simulink model "Cruise_control"  (R2018a)
settings: Solver=VariableStepAuto  StartTime=0.0  StopTime=10  MaxStep=0.01  RelTol=1e-4  EnableMultiTasking=on
values from neighbouring files (symbols this model uses):
  b_Ahead = 50    [ACC_DATA.m]    (also in CC_data.m)
  m_Ahead = 1000    [ACC_DATA.m]    (also in CC_data.m)
undefined symbols (not defined in the file or in its folder): b, m, sigbuilder_block
libraries: simulink x5
settings Model: Creator=Talha Rao  LastModifiedBy=Talha Rao
settings DataIOCC: LimitDataPoints=on  SaveOutput=off  SaveTime=off
settings OptimizationCC: ExpressionDepthLimit=2147483647  LifeSpan=1
settings DebuggingCC: UnderspecifiedInitializationDetection=Classic  MergeDetectMultiDrivingBlocksExec=none  FcnCallInpInsideContextMsg=warning  AllowSymbolicDim=off  StateNameClashWarn=warning  SFUnexpectedBacktrackingDiag=warning  SFNoUnconditionalDefaultTransitionDiag=warning  SFExecutionAtInitializationDiag=none
settings CodeAppCC: StateflowObjectComments=on
settings GRTTargetCC: TargetLangStandard=C89/C90 (ANSI)  GeneratePreprocessorConditionals=Disable all  CombineOutputUpdateFcns=off  GRTInterface=on

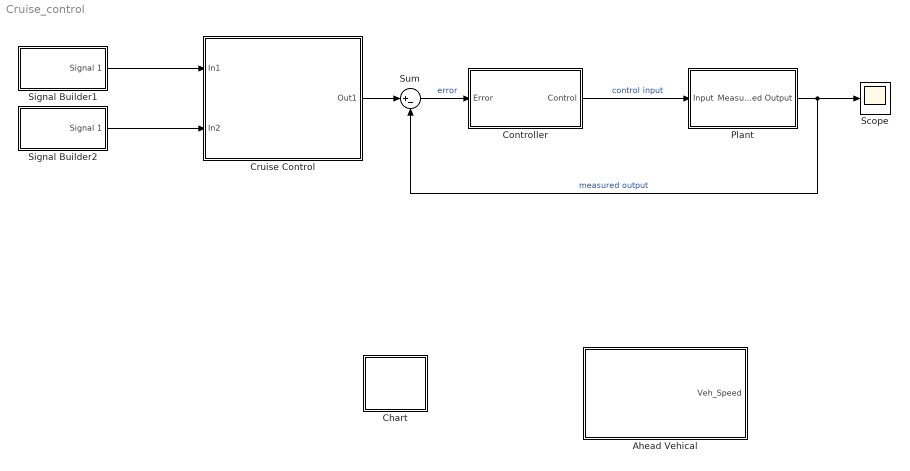
== system Cruise_control ==
  Ahead Vehical : Subsystem
      mask Display: image('C:\Users\Talha Rao\Pictures\index2 (2).jpg');
  Chart : Stateflow chart  TreatAsAtomicUnit=on
  Controller : Subsystem
  Cruise Control : Subsystem
  Plant : Subsystem
  Scope : Scope
  Signal Builder1 : Subsystem  Tag=STV Subsys  LoadFcn=sigbuilder_block('load');  StartFcn=sigbuilder_block('start');  StopFcn=sigbuilder_block('stop');  ClipboardFcn=sigbuilder_block('clipboard');  mask(Sigbuilder block){tuvar=[0:10]}
      mask help: Simulink:masks:SigbuilderBlock_MD
      mask init:
      | if ~strcmp(get_param(bdroot(gcbh),'SimulationStatus'),'stopped') tuvar = sigbuilder_block('maskInit'); end
      settings: CopyFcn=sigbuilder_block('copy');  DeleteFcn=sigbuilder_block('delete');  ModelCloseFcn=sigbuilder_block('modelClose');  PreSaveFcn=sigbuilder_block('preSave');  PauseFcn=sigbuilder_block('pause');  ContinueFcn=sigbuilder_block('continue');  NameChangeFcn=sigbuilder_block('namechange');  OpenFcn=sigbuilder_block('open',[437.6 199.2 550.4 400 ]);  CloseFcn=sigbuilder_block('close');
      mask Display: plot(0, 0, 100, 100,[2, 2, 32, 32, 2], [68, 8, 8, 68, 68],[32, 2], [38, 38], [32, 19, 2],[53, 60, 44], [32, 17, 17, 2],[16, 16, 31, 31]);txt = getActiveGroup(gcbh);text(2, 100, txt,'verticalAlignment', 'top');
  Signal Builder2 : Subsystem  Tag=STV Subsys  LoadFcn=sigbuilder_block('load');  StartFcn=sigbuilder_block('start');  StopFcn=sigbuilder_block('stop');  ClipboardFcn=sigbuilder_block('clipboard');  mask(Sigbuilder block){tuvar=[0:10]}
      mask help: Simulink:masks:SigbuilderBlock_MD
      mask init:
      | if ~strcmp(get_param(bdroot(gcbh),'SimulationStatus'),'stopped') tuvar = sigbuilder_block('maskInit'); end
      settings: CopyFcn=sigbuilder_block('copy');  DeleteFcn=sigbuilder_block('delete');  ModelCloseFcn=sigbuilder_block('modelClose');  PreSaveFcn=sigbuilder_block('preSave');  PauseFcn=sigbuilder_block('pause');  ContinueFcn=sigbuilder_block('continue');  NameChangeFcn=sigbuilder_block('namechange');  OpenFcn=sigbuilder_block('open',[437.6 199.2 550.4 400 ]);  CloseFcn=sigbuilder_block('close');
      mask Display: plot(0, 0, 100, 100,[2, 2, 32, 32, 2], [68, 8, 8, 68, 68],[32, 2], [38, 38], [32, 19, 2],[53, 60, 44], [32, 17, 17, 2],[16, 16, 31, 31]);txt = getActiveGroup(gcbh);text(2, 100, txt,'verticalAlignment', 'top');
  Sum : Sum  Inputs=|+-
  wires:
  Plant/1(Measured Output) -> Scope/1, Sum/2  "measured output"
  Sum/1 -> Controller/1(Error)  "error"
  Controller/1(Control) -> Plant/1(Input)  "control input"
  Signal Builder1/1(Signal 1) -> Cruise Control/1(In1)
  Signal Builder2/1(Signal 1) -> Cruise Control/2(In2)
  Cruise Control/1(Out1) -> Sum/1

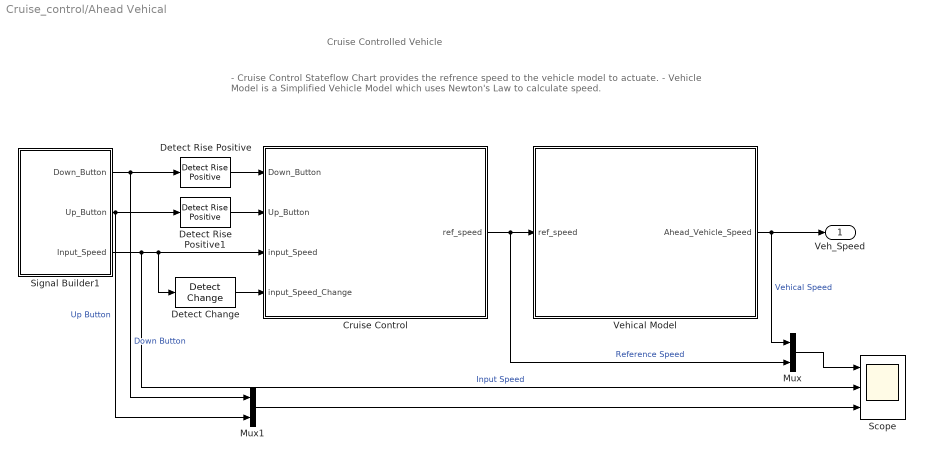
== system Cruise_control/Ahead Vehical ==
  note: - Cruise Control Stateflow Chart provides the refrence speed to the vehicle model to actuate.
      | - Vehicle Model is a Simplified Vehicle Model which uses Newton's Law to calculate speed.
  note: Cruise Controlled Vehicle
  Cruise Control : Stateflow chart  TreatAsAtomicUnit=on
  Detect Change : simulink/Logic and Bit Operations/Detect Change  vinit=0  OutDataTypeStr=boolean
  Detect Rise Positive : simulink/Logic and Bit Operations/Detect Rise Positive  vinit=0  OutDataTypeStr=boolean
  Detect Rise Positive1 : simulink/Logic and Bit Operations/Detect Rise Positive  vinit=0  OutDataTypeStr=boolean
  Mux : Mux  Inputs=2
  Mux1 : Mux  Inputs=2
  Scope : Scope  NumInputPorts=3
  Signal Builder1 : Subsystem  Tag=STV Subsys  LoadFcn=sigbuilder_block('load');  StartFcn=sigbuilder_block('start');  StopFcn=sigbuilder_block('stop');  ClipboardFcn=sigbuilder_block('clipboard');  mask(Sigbuilder block){tuvar=[0:10]}
      mask help: Simulink:masks:SigbuilderBlock_MD
      mask init:
      | if ~strcmp(get_param(bdroot(gcbh),'SimulationStatus'),'stopped') tuvar = sigbuilder_block('maskInit'); end
      settings: CopyFcn=sigbuilder_block('copy');  DeleteFcn=sigbuilder_block('delete');  ModelCloseFcn=sigbuilder_block('modelClose');  PreSaveFcn=sigbuilder_block('preSave');  PauseFcn=sigbuilder_block('pause');  ContinueFcn=sigbuilder_block('continue');  NameChangeFcn=sigbuilder_block('namechange');  OpenFcn=sigbuilder_block('open',[156 150.75 550.5 399.75 ]);  CloseFcn=sigbuilder_block('close');
      mask Display: plot(0, 0, 100, 100,[2, 2, 32, 32, 2], [68, 8, 8, 68, 68],[32, 2], [38, 38], [32, 19, 2],[53, 60, 44], [32, 17, 17, 2],[16, 16, 31, 31]);txt = getActiveGroup(gcbh);text(2, 100, txt,'verticalAlignment', 'top');
  Vehical Model : Subsystem
  Veh_Speed : Outport
  wires:
  Vehical Model/1(Ahead_Vehicle_Speed) -> Mux/1, Veh_Speed/1  "Vehical Speed"
  Detect Change/1 -> Cruise Control/4(input_Speed_Change)
  Cruise Control/1(ref_speed) -> Mux/2, Vehical Model/1(ref_speed)  "Reference Speed"
  Detect Rise Positive/1 -> Cruise Control/1(Down_Button)
  Signal Builder1/3(Input_Speed) -> Scope/2, Detect Change/1, Cruise Control/3(input_Speed)  "Input Speed"
  Signal Builder1/2(Up_Button) -> Detect Rise Positive1/1, Mux1/2  "Up Button"
  Signal Builder1/1(Down_Button) -> Mux1/1, Detect Rise Positive/1  "Down Button"
  Detect Rise Positive1/1 -> Cruise Control/2(Up_Button)
  Mux/1 -> Scope/1
  Mux1/1 -> Scope/3

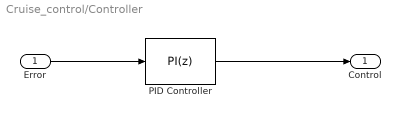
== system Cruise_control/Controller ==
  Error : Inport
  PID Controller : simulink/Continuous/PID Controller  Controller=PI  TimeDomain=Discrete-time  SampleTime=0.001  IntegratorMethod=Forward Euler  FilterMethod=Forward Euler  Form=Parallel  UseFilter=on  ControllerParametersSource=internal  P=392  I=19.5  D=0.02  N=20  InitialConditionSource=internal  InitialConditionForIntegrator=0  InitialConditionForFilter=0  ExternalReset=none  LimitOutput=off  UpperSaturationLimit=inf  LowerSaturationLimit=-inf  LinearizeAsGain=on  AntiWindupMode=none  Kb=1  TrackingMode=off  Kt=1  PParamMin=[]  PParamMax=[]  IParamMin=[]  IParamMax=[]  DParamMin=[]  DParamMax=[]  NParamMin=[]  NParamMax=[]  KbParamMin=[]  KbParamMax=[]  KtParamMin=[]  KtParamMax=[]  POutMin=[]  POutMax=[]  IOutMin=[]  IOutMax=[]  DOutMin=[]  DOutMax=[]  NOutMin=[]  NOutMax=[]  KbOutMin=[]  KbOutMax=[]  KtOutMin=[]  KtOutMax=[]  IntegratorOutMin=[]  IntegratorOutMax=[]  FilterOutMin=[]  FilterOutMax=[]  SumOutMin=[]  SumOutMax=[]  SumI1OutMin=[]  SumI1OutMax=[]  SumI2OutMin=[]  SumI2OutMax=[]  SumI3OutMin=[]  SumI3OutMax=[]  SumDOutMin=[]  SumDOutMax=[]  SaturationOutMin=[]  SaturationOutMax=[]  IntegratorContinuousStateAttributes=''  IntegratorStateMustResolveToSignalObject=off  IntegratorRTWStateStorageClass=Auto  FilterContinuousStateAttributes=''  FilterStateMustResolveToSignalObject=off  FilterRTWStateStorageClass=Auto  DifferentiatorICPrevScaledInput=0  DifferentiatorOutMin=[]  DifferentiatorOutMax=[]  FilterDiffOutCoefMin=[]  FilterDiffOutCoefMax=[]  SumDenOutMin=[]  SumDenOutMax=[]  SumNumOutMin=[]  SumNumOutMax=[]  ReciprocalOutMin=[]  ReciprocalOutMax=[]  DivideOutMin=[]  DivideOutMax=[]  TunerSelectOption=Transfer Function Based (PID Tuner App)
  Control : Outport
  wires:
  Error/1 -> PID Controller/1
  PID Controller/1 -> Control/1

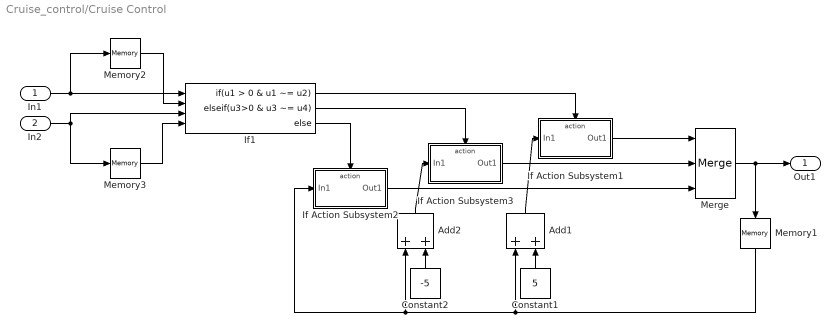
== system Cruise_control/Cruise Control ==
  In1 : Inport
  In2 : Inport  Port=2
  Add1 : Sum
  Add2 : Sum
  Constant1 : Constant  Value=5
  Constant2 : Constant  Value=-5
  If Action Subsystem1 : Subsystem  TreatAsAtomicUnit=on
  If Action Subsystem2 : Subsystem  TreatAsAtomicUnit=on
  If Action Subsystem3 : Subsystem  TreatAsAtomicUnit=on
  If1 : If  NumInputs=4  IfExpression=u1 > 0 & u1 ~= u2  ElseIfExpressions=u3>0 & u3 ~= u4
  Memory1 : Memory  InitialCondition=100
  Memory2 : Memory
  Memory3 : Memory
  Merge : Merge  Inputs=3
  Out1 : Outport
  wires:
  Merge/1 -> Out1/1, Memory1/1
  If1/1 -> If Action Subsystem1/Action
  If Action Subsystem1/1(Out1) -> Merge/1
  In2/1 -> Memory3/1, If1/3
  In1/1 -> Memory2/1, If1/1
  Constant1/1 -> Add1/2
  Memory2/1 -> If1/2
  If1/2 -> If Action Subsystem3/Action
  Memory1/1 -> If Action Subsystem2/1(In1), Add2/1, Add1/1
  Memory3/1 -> If1/4
  Add1/1 -> If Action Subsystem1/1(In1)
  Add2/1 -> If Action Subsystem3/1(In1)
  If1/3 -> If Action Subsystem2/Action
  Constant2/1 -> Add2/2
  If Action Subsystem2/1(Out1) -> Merge/3
  If Action Subsystem3/1(Out1) -> Merge/2

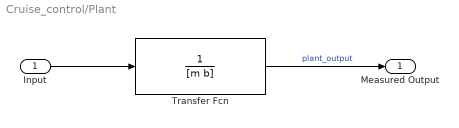
== system Cruise_control/Plant ==
  Input : Inport
  Transfer Fcn : TransferFcn  Denominator=[m b]
  Measured Output : Outport
  wires:
  Transfer Fcn/1 -> Measured Output/1  "plant_output"
  Input/1 -> Transfer Fcn/1

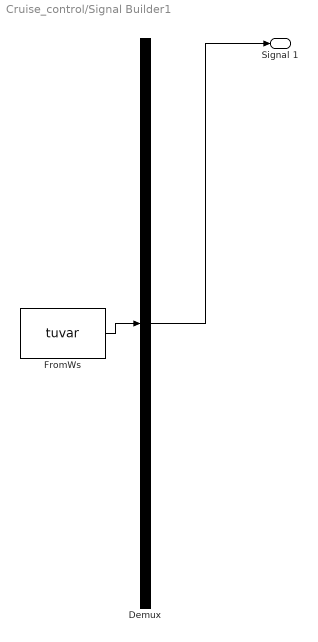
== system Cruise_control/Signal Builder1 ==
  Demux : Demux  Tag=STV Demux  Outputs=1
  FromWs : FromWorkspace  Tag=STV FromWs  VariableName=tuvar  SampleTime=0
      SigBuilderData=|
      | common.afterFinalStr = 'Extrapolate'
      | common.sampleTime = 0
      | dataSet.timeRange = [0 10]
      | dataSet.name = 'Group 1'
      | sbobj.Groups.Name = 'Group 1'
      | sbobj.Groups.Signals.Name = 'Signal 1'
      | sbobj.Groups.Signals.XData = [0 4 4 5 5 10]
      | sbobj.Groups.Signals.YData = [0 0 1 1 0 0]
  Signal 1 : Outport  Tag=STV Outport
  wires:
  Demux/1 -> Signal 1/1
  FromWs/1 -> Demux/1

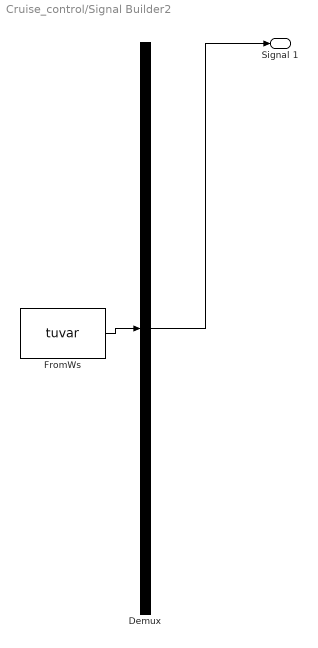
== system Cruise_control/Signal Builder2 ==
  Demux : Demux  Tag=STV Demux  Outputs=1
  FromWs : FromWorkspace  Tag=STV FromWs  VariableName=tuvar  SampleTime=0
      SigBuilderData=|
      | common.afterFinalStr = 'Extrapolate'
      | common.sampleTime = 0
      | dataSet.timeRange = [0 10]
      | dataSet.name = 'Group 1'
      | sbobj.Groups.Name = 'Group 1'
      | sbobj.Groups.Signals.Name = 'Signal 1'
      | sbobj.Groups.Signals.XData = [0 8 8 9 9 10]
      | sbobj.Groups.Signals.YData = [0 0 1 1 0 0]
  Signal 1 : Outport  Tag=STV Outport
  wires:
  Demux/1 -> Signal 1/1
  FromWs/1 -> Demux/1

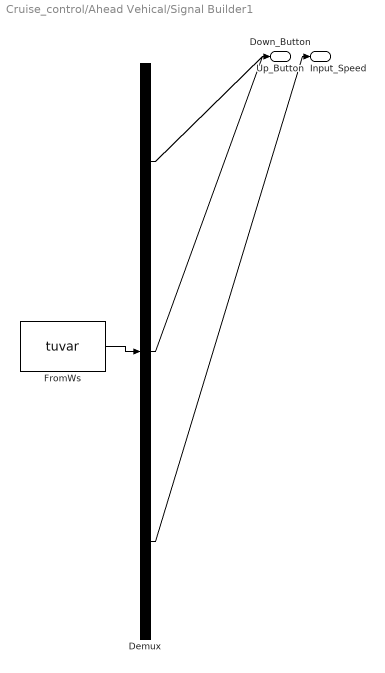
== system Cruise_control/Ahead Vehical/Signal Builder1 ==
  Demux : Demux  Tag=STV Demux  Outputs=3
  FromWs : FromWorkspace  Tag=STV FromWs  VariableName=tuvar  SampleTime=0
      SigBuilderData=|
      | common.afterFinalStr = 'Extrapolate'
      | common.sampleTime = 0
      | dataSet.timeRange = [0 200]
      | dataSet.name = 'Group 1'
      | sbobj.Groups.Name = 'Group 1'
      | sbobj.Groups.Signals(1).Name = 'Down_Button'
      | sbobj.Groups.Signals(1).XData = [0 90 90 92 92 100 100 102 102 150 150 152 152 200]
      | sbobj.Groups.Signals(1).YData = [0 0 1 1 0 0 1 1 0 0 1 1 0 0]
      | sbobj.Groups.Signals(2).Name = 'Up_Button'
      | sbobj.Groups.Signals(2).XData = [0 35 35 37 37 55 55 57 57 180 180 182 182 200]
      | sbobj.Groups.Signals(2).YData = [0 0 1 1 0 0 1 1 0 0 1 1 0 0]
      | sbobj.Groups.Signals(3).Name = 'Input_Speed'
      | sbobj.Groups.Signals(3).XData = [0 80 80 140 140 200]
      | sbobj.Groups.Signals(3).YData = [80 80 100 100 120 120]
      | sbobj.Groups.TimeRange = [0 200]
  Down_Button : Outport  Tag=STV Outport
  Up_Button : Outport  Tag=STV Outport  Port=2
  Input_Speed : Outport  Tag=STV Outport  Port=3
  wires:
  Demux/3 -> Input_Speed/1
  Demux/2 -> Up_Button/1
  Demux/1 -> Down_Button/1
  FromWs/1 -> Demux/1

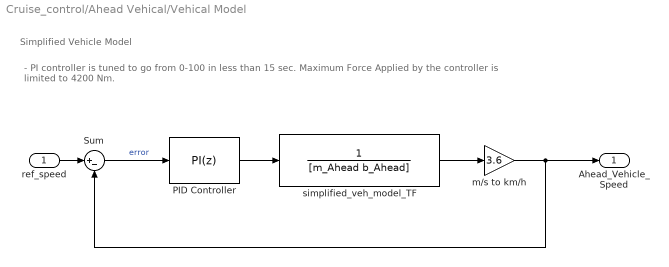
== system Cruise_control/Ahead Vehical/Vehical Model ==
  note: Simplified Vehicle Model
  note: - PI controller is tuned to go from 0-100 in less than 15 sec. Maximum Force Applied by the controller is limited to 4200 Nm.
  ref_speed : Inport
  PID Controller : simulink/Continuous/PID Controller  Controller=PI  TimeDomain=Discrete-time  SampleTime=0.001  IntegratorMethod=Forward Euler  FilterMethod=Forward Euler  Form=Parallel  UseFilter=on  ControllerParametersSource=internal  P=125  I=7.2  D=0.02  N=20  InitialConditionSource=internal  InitialConditionForIntegrator=0  InitialConditionForFilter=0  ExternalReset=none  LimitOutput=on  UpperSaturationLimit=4200  LowerSaturationLimit=0  LinearizeAsGain=on  AntiWindupMode=none  Kb=1  TrackingMode=off  Kt=1  PParamMin=[]  PParamMax=[]  IParamMin=[]  IParamMax=[]  DParamMin=[]  DParamMax=[]  NParamMin=[]  NParamMax=[]  KbParamMin=[]  KbParamMax=[]  KtParamMin=[]  KtParamMax=[]  POutMin=[]  POutMax=[]  IOutMin=[]  IOutMax=[]  DOutMin=[]  DOutMax=[]  NOutMin=[]  NOutMax=[]  KbOutMin=[]  KbOutMax=[]  KtOutMin=[]  KtOutMax=[]  IntegratorOutMin=[]  IntegratorOutMax=[]  FilterOutMin=[]  FilterOutMax=[]  SumOutMin=[]  SumOutMax=[]  SumI1OutMin=[]  SumI1OutMax=[]  SumI2OutMin=[]  SumI2OutMax=[]  SumI3OutMin=[]  SumI3OutMax=[]  SumDOutMin=[]  SumDOutMax=[]  SaturationOutMin=[]  SaturationOutMax=[]  IntegratorContinuousStateAttributes=''  IntegratorStateMustResolveToSignalObject=off  IntegratorRTWStateStorageClass=Auto  FilterContinuousStateAttributes=''  FilterStateMustResolveToSignalObject=off  FilterRTWStateStorageClass=Auto  DifferentiatorICPrevScaledInput=0  DifferentiatorOutMin=[]  DifferentiatorOutMax=[]  FilterDiffOutCoefMin=[]  FilterDiffOutCoefMax=[]  SumDenOutMin=[]  SumDenOutMax=[]  SumNumOutMin=[]  SumNumOutMax=[]  ReciprocalOutMin=[]  ReciprocalOutMax=[]  DivideOutMin=[]  DivideOutMax=[]  TunerSelectOption=Transfer Function Based (PID Tuner App)
  Sum : Sum  Inputs=|+-
  m/s to km/h : Gain  Gain=3.6
  simplified_veh_model_TF : TransferFcn  Denominator=[m_Ahead b_Ahead]
  Ahead_Vehicle_Speed : Outport
  wires:
  ref_speed/1 -> Sum/1
  Sum/1 -> PID Controller/1  "error"
  m/s to km/h/1 -> Sum/2, Ahead_Vehicle_Speed/1
  simplified_veh_model_TF/1 -> m/s to km/h/1
  PID Controller/1 -> simplified_veh_model_TF/1

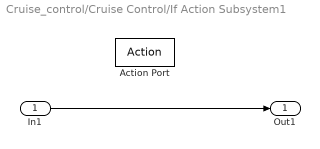
== system Cruise_control/Cruise Control/If Action Subsystem1 ==
  In1 : Inport
  Action Port : ActionPort  ActionType=then
  Out1 : Outport
  wires:
  In1/1 -> Out1/1

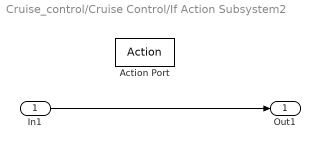
== system Cruise_control/Cruise Control/If Action Subsystem2 ==
  In1 : Inport
  Action Port : ActionPort  ActionType=else
  Out1 : Outport
  wires:
  In1/1 -> Out1/1

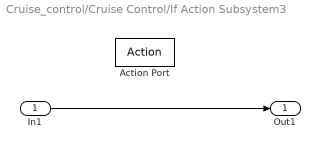
== system Cruise_control/Cruise Control/If Action Subsystem3 ==
  In1 : Inport
  Action Port : ActionPort  ActionType=elseif
  Out1 : Outport
  wires:
  In1/1 -> Out1/1

== stateflow chart Cruise_control/Ahead Vehical/Cruise Control ==
  note: Cruise Control
  note: State
      | Description
      | Condition
      | Next State
      |
      | CRUISE_ONTROL_ON
      | Default State where ref_speed is initially set to input speed
      | Default
      | UP_BUTTON_PRESSED / DOWN_BUTTON_PRESSED /
      | REFRESH_TO_REFRENCE
      |
      | UP_BUTTON_PRESSED
      | If the up button is pressed, increase speed by 5 km/h and return to default state immediately.
      | UP_BUTTON is pressed
      | CRUISE_ONTROL_ON
      |
      | DOWN_BUTTON_PRESSED
      | If the down button is pressed, decrease speed by 5 km/h and return to default state immediately.
      | DOWN_BUTTON is pressed
      | CRUISE_ONTROL_ON
      |
      | REFRESH_TO_REFRENCE
      | If system detects a change in input speed, overrule the previous refrence speed and adjust to the new input speed. Leaves the state if refrence speed becomes equal to input speed
      | Input Speed is changed
      | CRUISE_ONTROL_ON
  state UP_BUTTON_PRESSED
    ref_speed = ref_speed + 5;
  state DOWN_BUTTON_PRESSED
    ref_speed = ref_speed - 5;
  state CRUISE_ONTROL_ON
    ref_speed = ref_speed;
  state REFRESH_TO_REFRENCE
    ref_speed = input_Speed;
  (default) -> CRUISE_ONTROL_ON : {ref_speed = input_Speed}
  CRUISE_ONTROL_ON -> DOWN_BUTTON_PRESSED [order 2] : [Down_Button>0]
  CRUISE_ONTROL_ON -> UP_BUTTON_PRESSED [order 1] : [Up_Button > 0]
  DOWN_BUTTON_PRESSED -> CRUISE_ONTROL_ON
  UP_BUTTON_PRESSED -> CRUISE_ONTROL_ON
  REFRESH_TO_REFRENCE -> CRUISE_ONTROL_ON : [input_Speed == ref_speed]
  CRUISE_ONTROL_ON -> REFRESH_TO_REFRENCE [order 3] : [input_Speed_Change > 0]
  data: Down_Button input; Up_Button input; input_Speed input; input_Speed_Change input; ref_speed output

== stateflow chart Cruise_control/Chart ==
  (default) -> (junction 1)
